simulink model "ILIAD_setup"  (R2017a)
settings: Solver=FixedStepDiscrete  StartTime=0.0  StopTime=running_time  FixedStep=0.01  RelTol=1e-3  EnableMultiTasking=on
undefined symbols (not defined in the file or in its folder): Orientation, Position
libraries: robotlib x8, QB_pacer_lib x1
settings Model: Creator=Eng  LastModifiedBy=ale
settings DataIOCC: LimitDataPoints=on  SaveFormat=Array
settings OptimizationCC: LifeSpan=inf
settings DebuggingCC: UnderspecifiedInitializationDetection=Classic  MergeDetectMultiDrivingBlocksExec=none  SolverPrmCheckMsg=warning  SFUnexpectedBacktrackingDiag=warning  SFNoUnconditionalDefaultTransitionDiag=warning  SFExecutionAtInitializationDiag=none
settings HardwareCC: ProdBitPerPointer=32  ProdBitPerSizeT=32  ProdBitPerPtrDiffT=32  ProdLargestAtomicFloat=None  ProdIntDivRoundTo=Undefined  ProdEndianess=Unspecified  ProdWordSize=32  ProdHWDeviceType=32-bit Generic
settings ModelReferenceCC: PropagateSignalLabelsOutOfModel=off
settings GRTTargetCC: TargetLangStandard=C89/C90 (ANSI)  GeneratePreprocessorConditionals=Disable all
settings ConfigComp: CovMetricSettings=dw  CovHtmlReporting=on  CovSaveCumulativeToWorkspaceVar=on  CovSaveSingleToWorkspaceVar=on  CovExternalEMLEnable=off

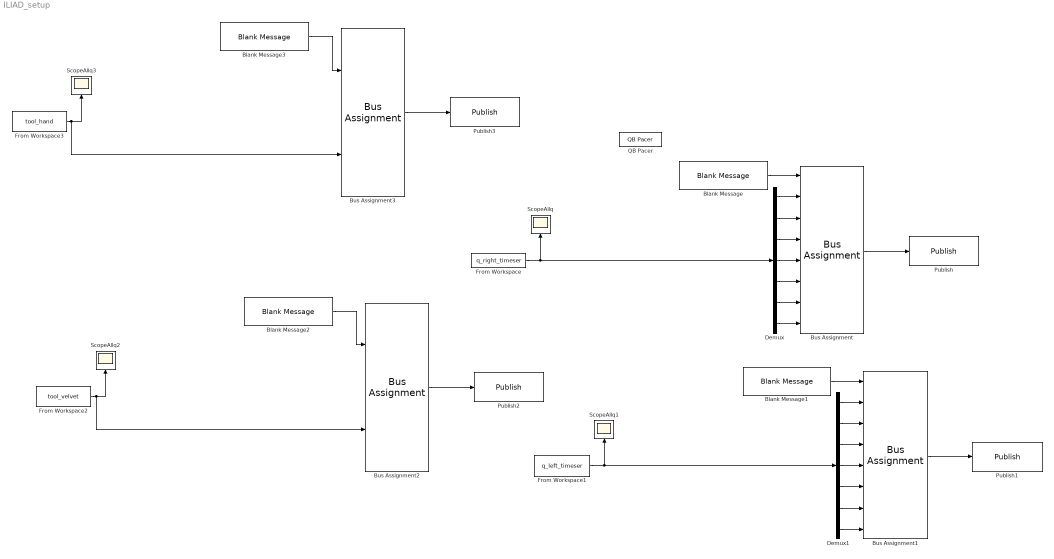
== system ILIAD_setup ==
  Blank Message : robotlib/Blank Message  SourceLibraryInfo=This block requires Robotics System Toolbox  messageType=geometry_msgs/Pose  SampleTime=inf
      settings: SourceProductBaseCode=RO
  Blank Message1 : robotlib/Blank Message  SourceLibraryInfo=This block requires Robotics System Toolbox  messageType=geometry_msgs/Pose  SampleTime=inf
      settings: SourceProductBaseCode=RO
  Blank Message2 : robotlib/Blank Message  SourceLibraryInfo=This block requires Robotics System Toolbox  messageType=std_msgs/Float64  SampleTime=inf
      settings: SourceProductBaseCode=RO
  Blank Message3 : robotlib/Blank Message  SourceLibraryInfo=This block requires Robotics System Toolbox  messageType=std_msgs/Float64  SampleTime=inf
      settings: SourceProductBaseCode=RO
  Bus Assignment : BusAssignment  AssignedSignals=Position.X,Position.Y,Position.Z,Orientation.X,Orientation.Y,Orientation.Z,Orientation.W
  Bus Assignment1 : BusAssignment  AssignedSignals=Position.X,Position.Y,Position.Z,Orientation.X,Orientation.Y,Orientation.Z,Orientation.W
  Bus Assignment2 : BusAssignment  AssignedSignals=Data
  Bus Assignment3 : BusAssignment  AssignedSignals=Data
  Demux : Demux  Outputs=7
  Demux1 : Demux  Outputs=7
  From Workspace : FromWorkspace  VariableName=q_right_timeser  SampleTime=0
  From Workspace1 : FromWorkspace  VariableName=q_left_timeser  SampleTime=0
  From Workspace2 : FromWorkspace  VariableName=tool_velvet  SampleTime=0
  From Workspace3 : FromWorkspace  VariableName=tool_hand  SampleTime=0
  Publish : robotlib/Publish  SourceLibraryInfo=This block requires Robotics System Toolbox  topicSource=Specify your own  topic=/matlab_right  messageType=geometry_msgs/Pose  messageQueueLength=1
      settings: SourceProductBaseCode=RO
  Publish1 : robotlib/Publish  SourceLibraryInfo=This block requires Robotics System Toolbox  topicSource=Specify your own  topic=/matlab_left  messageType=geometry_msgs/Pose  messageQueueLength=1
      settings: SourceProductBaseCode=RO
  Publish2 : robotlib/Publish  SourceLibraryInfo=This block requires Robotics System Toolbox  topicSource=Select from ROS network  topic=/velvet_cmd  messageType=std_msgs/Float64  messageQueueLength=1
      settings: SourceProductBaseCode=RO
  Publish3 : robotlib/Publish  SourceLibraryInfo=This block requires Robotics System Toolbox  topicSource=Select from ROS network  topic=/hand_cmd  messageType=std_msgs/Float64  messageQueueLength=1
      settings: SourceProductBaseCode=RO
  QB Pacer : QB_pacer_lib/QB Pacer  simTimePerRealTime=1
  ScopeAllq{,1..3} (4 alike) : Scope
  wires:
  From Workspace/1 -> ScopeAllq/1, Demux/1
  Bus Assignment/1 -> Publish/1
  Blank Message/1 -> Bus Assignment/1
  Demux/1 -> Bus Assignment/2
  Demux/3 -> Bus Assignment/4
  Demux/4 -> Bus Assignment/5
  Demux/2 -> Bus Assignment/3
  Demux/6 -> Bus Assignment/7
  Demux/5 -> Bus Assignment/6
  Demux/7 -> Bus Assignment/8
  From Workspace1/1 -> ScopeAllq1/1, Demux1/1
  Bus Assignment1/1 -> Publish1/1
  Demux1/1 -> Bus Assignment1/2
  Demux1/3 -> Bus Assignment1/4
  Demux1/4 -> Bus Assignment1/5
  Demux1/2 -> Bus Assignment1/3
  Demux1/6 -> Bus Assignment1/7
  Demux1/5 -> Bus Assignment1/6
  Demux1/7 -> Bus Assignment1/8
  Blank Message1/1 -> Bus Assignment1/1
  From Workspace2/1 -> Bus Assignment2/2, ScopeAllq2/1
  Bus Assignment2/1 -> Publish2/1
  Blank Message2/1 -> Bus Assignment2/1
  From Workspace3/1 -> Bus Assignment3/2, ScopeAllq3/1
  Bus Assignment3/1 -> Publish3/1
  Blank Message3/1 -> Bus Assignment3/1
